simulink model "gm_N4"  (R2016b)
settings: Solver=FixedStepDiscrete  StartTime=0.0  StopTime=10.0  RelTol=1e-3
libraries: simulink x12
settings Model: Creator=hasee  LastModifiedBy=hasee
settings DataIOCC: LimitDataPoints=on  SaveOutput=off  SaveTime=off
settings OptimizationCC: BlockReduction=off  ConditionallyExecuteInputs=off  DefaultParameterBehavior=Inlined  LifeSpan=inf
settings DebuggingCC: AlgebraicLoopMsg=error  InheritedTsInSrcMsg=none  SingleTaskRateTransMsg=error  AllowSymbolicDim=off  StrictBusMsg=ErrorOnBusTreatedAsVector  SFUnexpectedBacktrackingDiag=warning  SFNoUnconditionalDefaultTransitionDiag=warning  SFExecutionAtInitializationDiag=none
settings HardwareCC: ProdBitPerPointer=32  ProdBitPerSizeT=32  ProdBitPerPtrDiffT=32  ProdLargestAtomicFloat=None  ProdIntDivRoundTo=Undefined  ProdEndianess=Unspecified  ProdWordSize=32  ProdHWDeviceType=ASIC/FPGA->ASIC/FPGA  ProdEqTarget=off
settings GRTTargetCC: TargetLangStandard=C89/C90 (ANSI)  GeneratePreprocessorConditionals=Disable all
settings ConfigComp: CovScope=ReferencedModels  CovMetricSettings=dw  CovHtmlReporting=on  CovSaveCumulativeToWorkspaceVar=on  CovSaveSingleToWorkspaceVar=on  CovExternalEMLEnable=off  CovSFcnEnable=off

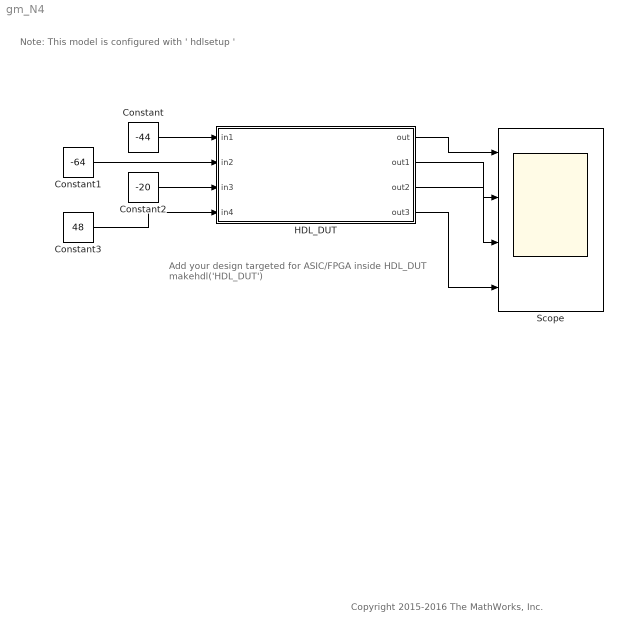
== system gm_N4 ==
  note: Copyright 2015-2016 The MathWorks, Inc.
  note: Add your design targeted for ASIC/FPGA inside HDL_DUT
      | makehdl('HDL_DUT')
  note: Note: This model is configured with ' hdlsetup '
  Constant : Constant  Value=-44  OutDataTypeStr=int8  SampleTime=-1
  Constant1 : Constant  Value=-64  OutDataTypeStr=int8  SampleTime=-1
  Constant2 : Constant  Value=-20  OutDataTypeStr=int8  SampleTime=-1
  Constant3 : Constant  Value=48  OutDataTypeStr=int8  SampleTime=-1
  HDL_DUT : Subsystem
  Scope : Scope  NumInputPorts=4
  wires:
  Constant2/1 -> HDL_DUT/3(in3)
  Constant3/1 -> HDL_DUT/4(in4)
  Constant1/1 -> HDL_DUT/2(in2)
  HDL_DUT/4(out3) -> Scope/4
  HDL_DUT/3(out2) -> Scope/3
  HDL_DUT/2(out1) -> Scope/2
  HDL_DUT/1(out) -> Scope/1
  Constant/1 -> HDL_DUT/1(in1)

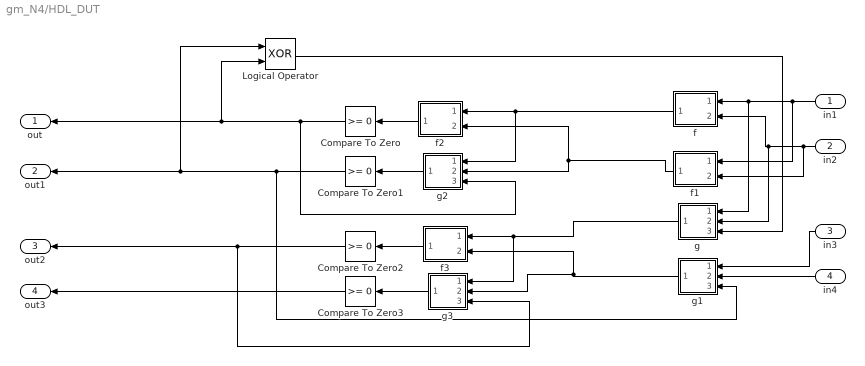
== system gm_N4/HDL_DUT ==
  in1 : Inport
  in2 : Inport  Port=2
  in3 : Inport  Port=3
  in4 : Inport  Port=4
  Compare To Zero{,1..3} (4 alike) : simulink/Logic and Bit Operations/Compare To Zero  relop=>=  OutDataTypeStr=boolean
  Logical Operator : Logic  Operator=XOR  AllPortsSameDT=off  OutDataTypeStr=boolean
  f : Subsystem
  f1 : Subsystem
  f2 : Subsystem
  f3 : Subsystem
  g : Subsystem
  g1 : Subsystem
  g2 : Subsystem
  g3 : Subsystem
  out : Outport
  out1 : Outport  Port=2
  out2 : Outport  Port=3
  out3 : Outport  Port=4
  wires:
  Compare To Zero3/1 -> out3/1
  g3/1(out) -> Compare To Zero3/1
  Compare To Zero2/1 -> out2/1, g3/3(in3)
  g1/1(out) -> f3/2(in2), g3/2(in2)
  g/1(out) -> f3/1(in1), g3/1(in1)
  f3/1(out1) -> Compare To Zero2/1
  in4/1 -> g1/2(in2)
  in3/1 -> g1/1(in1)
  Logical Operator/1 -> g/3(in3)
  Compare To Zero1/1 -> out1/1, Logical Operator/1, g1/3(in3)
  g2/1(out) -> Compare To Zero1/1
  Compare To Zero/1 -> out/1, Logical Operator/2, g2/3(in3)
  f2/1(out1) -> Compare To Zero/1
  f1/1(out1) -> f2/2(in2), g2/2(in2)
  f/1(out1) -> f2/1(in1), g2/1(in1)
  in2/1 -> f/2(in2), g/2(in2), f1/2(in2)
  in1/1 -> f/1(in1), g/1(in1), f1/1(in1)

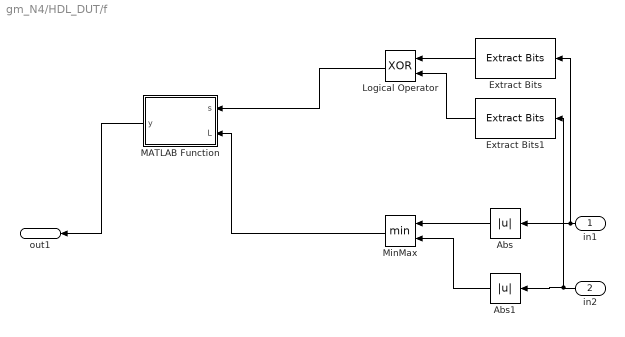
== system gm_N4/HDL_DUT/f ==
  in1 : Inport  OutDataTypeStr=int8
  in2 : Inport  Port=2  OutDataTypeStr=int8
  Abs : Abs
  Abs1 : Abs
  Extract Bits : simulink/Logic and Bit Operations/Extract Bits  bitsToExtract=Range starting with most significant bit  numBits=1  bitIdxRange=[0 ]  outScalingMode=Preserve fixed-point scaling
  Extract Bits1 : simulink/Logic and Bit Operations/Extract Bits  bitsToExtract=Range starting with most significant bit  numBits=1  bitIdxRange=[0 ]  outScalingMode=Preserve fixed-point scaling
  Logical Operator : Logic  Operator=XOR  AllPortsSameDT=off  OutDataTypeStr=boolean
  MATLAB Function : MATLAB Function  TreatAsAtomicUnit=on
  MinMax : MinMax  Inputs=2
  out1 : Outport
  wires:
  MATLAB Function/1(y) -> out1/1
  MinMax/1 -> MATLAB Function/2(L)
  Abs1/1 -> MinMax/2
  Abs/1 -> MinMax/1
  Logical Operator/1 -> MATLAB Function/1(s)
  Extract Bits1/1 -> Logical Operator/2
  in2/1 -> Extract Bits1/1, Abs1/1
  in1/1 -> Extract Bits/1, Abs/1
  Extract Bits/1 -> Logical Operator/1

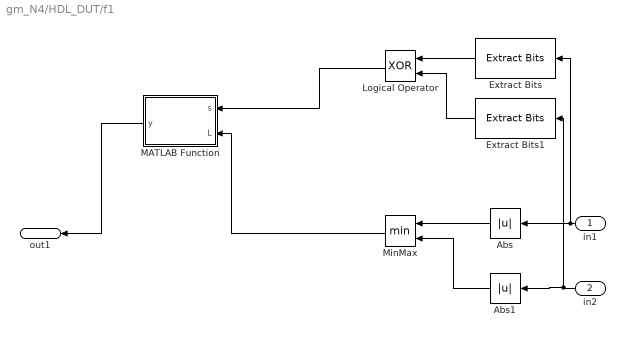
== system gm_N4/HDL_DUT/f1 ==
  in1 : Inport  OutDataTypeStr=int8
  in2 : Inport  Port=2  OutDataTypeStr=int8
  Abs : Abs
  Abs1 : Abs
  Extract Bits : simulink/Logic and Bit Operations/Extract Bits  bitsToExtract=Range starting with most significant bit  numBits=1  bitIdxRange=[0 ]  outScalingMode=Preserve fixed-point scaling
  Extract Bits1 : simulink/Logic and Bit Operations/Extract Bits  bitsToExtract=Range starting with most significant bit  numBits=1  bitIdxRange=[0 ]  outScalingMode=Preserve fixed-point scaling
  Logical Operator : Logic  Operator=XOR  AllPortsSameDT=off  OutDataTypeStr=boolean
  MATLAB Function : MATLAB Function  TreatAsAtomicUnit=on
  MinMax : MinMax  Inputs=2
  out1 : Outport
  wires:
  MATLAB Function/1(y) -> out1/1
  MinMax/1 -> MATLAB Function/2(L)
  Abs1/1 -> MinMax/2
  Abs/1 -> MinMax/1
  Logical Operator/1 -> MATLAB Function/1(s)
  Extract Bits1/1 -> Logical Operator/2
  in2/1 -> Extract Bits1/1, Abs1/1
  in1/1 -> Extract Bits/1, Abs/1
  Extract Bits/1 -> Logical Operator/1

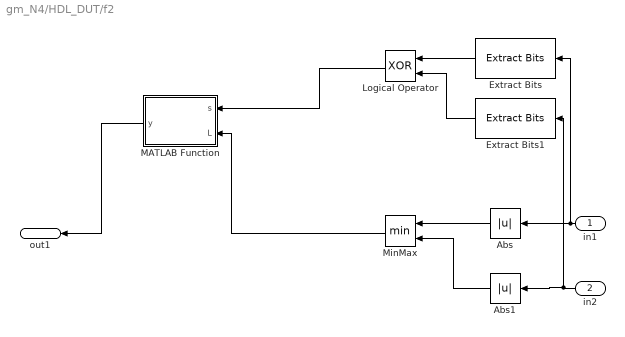
== system gm_N4/HDL_DUT/f2 ==
  in1 : Inport  OutDataTypeStr=int8
  in2 : Inport  Port=2  OutDataTypeStr=int8
  Abs : Abs
  Abs1 : Abs
  Extract Bits : simulink/Logic and Bit Operations/Extract Bits  bitsToExtract=Range starting with most significant bit  numBits=1  bitIdxRange=[0 ]  outScalingMode=Preserve fixed-point scaling
  Extract Bits1 : simulink/Logic and Bit Operations/Extract Bits  bitsToExtract=Range starting with most significant bit  numBits=1  bitIdxRange=[0 ]  outScalingMode=Preserve fixed-point scaling
  Logical Operator : Logic  Operator=XOR  AllPortsSameDT=off  OutDataTypeStr=boolean
  MATLAB Function : MATLAB Function  TreatAsAtomicUnit=on
  MinMax : MinMax  Inputs=2
  out1 : Outport
  wires:
  MATLAB Function/1(y) -> out1/1
  MinMax/1 -> MATLAB Function/2(L)
  Abs1/1 -> MinMax/2
  Abs/1 -> MinMax/1
  Logical Operator/1 -> MATLAB Function/1(s)
  Extract Bits1/1 -> Logical Operator/2
  in2/1 -> Extract Bits1/1, Abs1/1
  in1/1 -> Extract Bits/1, Abs/1
  Extract Bits/1 -> Logical Operator/1

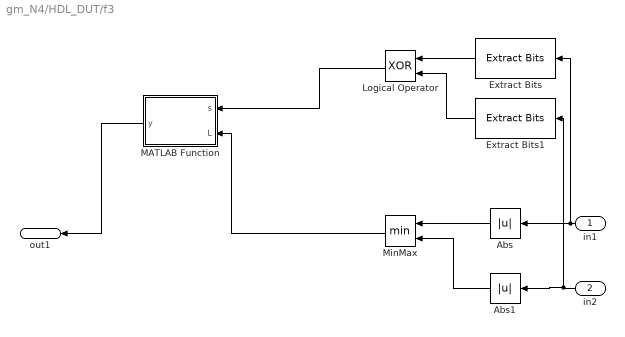
== system gm_N4/HDL_DUT/f3 ==
  in1 : Inport  OutDataTypeStr=int8
  in2 : Inport  Port=2  OutDataTypeStr=int8
  Abs : Abs
  Abs1 : Abs
  Extract Bits : simulink/Logic and Bit Operations/Extract Bits  bitsToExtract=Range starting with most significant bit  numBits=1  bitIdxRange=[0 ]  outScalingMode=Preserve fixed-point scaling
  Extract Bits1 : simulink/Logic and Bit Operations/Extract Bits  bitsToExtract=Range starting with most significant bit  numBits=1  bitIdxRange=[0 ]  outScalingMode=Preserve fixed-point scaling
  Logical Operator : Logic  Operator=XOR  AllPortsSameDT=off  OutDataTypeStr=boolean
  MATLAB Function : MATLAB Function  TreatAsAtomicUnit=on
  MinMax : MinMax  Inputs=2
  out1 : Outport
  wires:
  MATLAB Function/1(y) -> out1/1
  MinMax/1 -> MATLAB Function/2(L)
  Abs1/1 -> MinMax/2
  Abs/1 -> MinMax/1
  Logical Operator/1 -> MATLAB Function/1(s)
  Extract Bits1/1 -> Logical Operator/2
  in2/1 -> Extract Bits1/1, Abs1/1
  in1/1 -> Extract Bits/1, Abs/1
  Extract Bits/1 -> Logical Operator/1

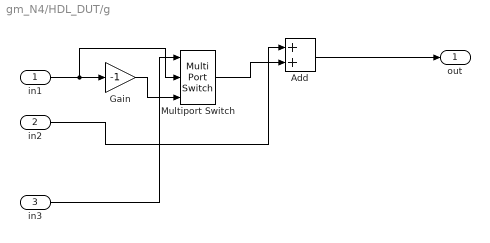
== system gm_N4/HDL_DUT/g ==
  in1 : Inport
  in2 : Inport  Port=2
  in3 : Inport  Port=3  OutDataTypeStr=boolean
  Add : Sum  Inputs=2  AccumDataTypeStr=int8
  Gain : Gain  Gain=-1  OutDataTypeStr=int8
  Multiport Switch : MultiPortSwitch  DataPortOrder=Zero-based contiguous  Inputs=2  OutDataTypeStr=int8
  out : Outport
  wires:
  Add/1 -> out/1
  Multiport Switch/1 -> Add/2
  in2/1 -> Add/1
  Gain/1 -> Multiport Switch/3
  in3/1 -> Multiport Switch/1
  in1/1 -> Gain/1, Multiport Switch/2

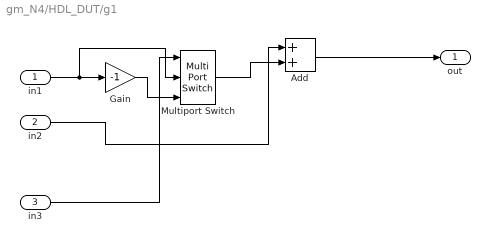
== system gm_N4/HDL_DUT/g1 ==
  in1 : Inport
  in2 : Inport  Port=2
  in3 : Inport  Port=3  OutDataTypeStr=boolean
  Add : Sum  Inputs=2  AccumDataTypeStr=int8
  Gain : Gain  Gain=-1  OutDataTypeStr=int8
  Multiport Switch : MultiPortSwitch  DataPortOrder=Zero-based contiguous  Inputs=2  OutDataTypeStr=int8
  out : Outport
  wires:
  Add/1 -> out/1
  Multiport Switch/1 -> Add/2
  in2/1 -> Add/1
  Gain/1 -> Multiport Switch/3
  in3/1 -> Multiport Switch/1
  in1/1 -> Gain/1, Multiport Switch/2

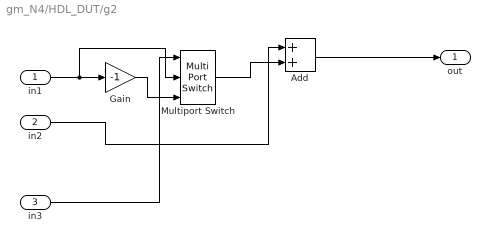
== system gm_N4/HDL_DUT/g2 ==
  in1 : Inport
  in2 : Inport  Port=2
  in3 : Inport  Port=3  OutDataTypeStr=boolean
  Add : Sum  Inputs=2  AccumDataTypeStr=int8
  Gain : Gain  Gain=-1  OutDataTypeStr=int8
  Multiport Switch : MultiPortSwitch  DataPortOrder=Zero-based contiguous  Inputs=2  OutDataTypeStr=int8
  out : Outport
  wires:
  Add/1 -> out/1
  Multiport Switch/1 -> Add/2
  in2/1 -> Add/1
  Gain/1 -> Multiport Switch/3
  in3/1 -> Multiport Switch/1
  in1/1 -> Gain/1, Multiport Switch/2

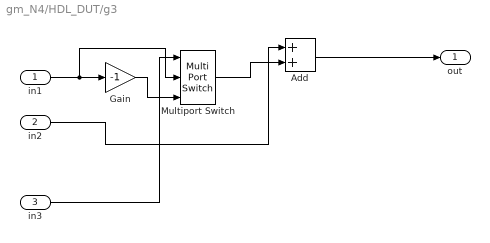
== system gm_N4/HDL_DUT/g3 ==
  in1 : Inport
  in2 : Inport  Port=2
  in3 : Inport  Port=3  OutDataTypeStr=boolean
  Add : Sum  Inputs=2  AccumDataTypeStr=int8
  Gain : Gain  Gain=-1  OutDataTypeStr=int8
  Multiport Switch : MultiPortSwitch  DataPortOrder=Zero-based contiguous  Inputs=2  OutDataTypeStr=int8
  out : Outport
  wires:
  Add/1 -> out/1
  Multiport Switch/1 -> Add/2
  in2/1 -> Add/1
  Gain/1 -> Multiport Switch/3
  in3/1 -> Multiport Switch/1
  in1/1 -> Gain/1, Multiport Switch/2

== matlab function gm_N4/HDL_DUT/f/MATLAB Function ==
  data: s input; y output; L input
function y = fcn(s,L)
%#codegen
if s ==1
    y = -L;
else
    y = L;
end

== matlab function gm_N4/HDL_DUT/f1/MATLAB Function ==
  data: s input; y output; L input
function y = fcn(s,L)
%#codegen
if s ==1
    y = -L;
else
    y = L;
end

== matlab function gm_N4/HDL_DUT/f2/MATLAB Function ==
  data: s input; y output; L input
function y = fcn(s,L)
%#codegen
if s ==1
    y = -L;
else
    y = L;
end

== matlab function gm_N4/HDL_DUT/f3/MATLAB Function ==
  data: s input; y output; L input
function y = fcn(s,L)
%#codegen
if s ==1
    y = -L;
else
    y = L;
end
